simulink model "c00015M_harness"  (R2018a)
settings: Solver=FixedStepAuto  StartTime=0.0  StopTime=300  FixedStep=0.1  RelTol=1e-3
undefined symbols (not defined in the file): A1, hmax, PriorityTank, R1, R2, sigbuilder_block, TempThreshold
(part 9 of 33)

== system c00015M_harness/M078/Tank3 ==
  CT3 : Inport
  T3 : Inport  Port=2
  EB3 : Inport  Port=3
  LL1 : Inport  Port=4
  Control : Subsystem
  Logical Operator : Logic  AllPortsSameDT=off  OutDataTypeStr=boolean
  MasterTankControl : Subsystem
  Memory : Memory
  Memory1 : Memory
  TankModel : Subsystem
  LL3 : Outport
  wires:
  TankModel/1(LiquidLevel) -> Memory/1, LL3/1
  Control/1(LiquidIn) -> Logical Operator/1
  Control/2(LiquidOut) -> TankModel/2(LiquidOut)
  Memory/1 -> MasterTankControl/2(LiquidTank3), Control/5(LiquidLevel)
  CT3/1 -> Control/2(StartMaintenance), Control/1(ControlType)
  Memory1/1 -> MasterTankControl/1(LiquidTank1)
  EB3/1 -> Control/3(EmergencyButton)
  MasterTankControl/1(AllowTheTankFilling) -> Logical Operator/2
  Logical Operator/1 -> TankModel/1(LiquidIn)
  LL1/1 -> Memory1/1
  T3/1 -> Control/4(Temperature)

== system c00015M_harness/M079/Tank1 ==
  CT1 : Inport
  T1 : Inport  Port=2
  EB1 : Inport  Port=3
  LL3 : Inport  Port=4
  Control : Subsystem
  Logical Operator : Logic  AllPortsSameDT=off  OutDataTypeStr=boolean
  MasterTankControl : Subsystem
  Memory : Memory
  Memory2 : Memory
  TankModel : Subsystem
  LL1 : Outport
  wires:
  TankModel/1(LiquidLevel) -> Memory/1, LL1/1
  Control/1(LiquidIn) -> Logical Operator/1
  Control/2(LiquidOut) -> TankModel/2(LiquidOut)
  Memory/1 -> Control/5(LiquidLevel), MasterTankControl/1(LiquidTank1)
  CT1/1 -> Control/2(StartMaintenance), Control/1(ControlType)
  LL3/1 -> Memory2/1
  Memory2/1 -> MasterTankControl/2(LiquidTank3)
  EB1/1 -> Control/3(EmergencyButton)
  MasterTankControl/1(AllowTheTankFilling) -> Logical Operator/2
  Logical Operator/1 -> TankModel/1(LiquidIn)
  T1/1 -> Control/4(Temperature)

== system c00015M_harness/M079/Tank3 ==
  CT3 : Inport
  T3 : Inport  Port=2
  EB3 : Inport  Port=3
  LL1 : Inport  Port=4
  Control : Subsystem
  Logical Operator : Logic  AllPortsSameDT=off  OutDataTypeStr=boolean
  MasterTankControl : Subsystem
  Memory : Memory
  Memory1 : Memory
  TankModel : Subsystem
  LL3 : Outport
  wires:
  TankModel/1(LiquidLevel) -> Memory/1, LL3/1
  Control/1(LiquidIn) -> Logical Operator/1
  Control/2(LiquidOut) -> TankModel/2(LiquidOut)
  Memory/1 -> MasterTankControl/2(LiquidTank3), Control/5(LiquidLevel)
  CT3/1 -> Control/2(StartMaintenance), Control/1(ControlType)
  Memory1/1 -> MasterTankControl/1(LiquidTank1)
  EB3/1 -> Control/3(EmergencyButton)
  MasterTankControl/1(AllowTheTankFilling) -> Logical Operator/2
  Logical Operator/1 -> TankModel/1(LiquidIn)
  LL1/1 -> Memory1/1
  T3/1 -> Control/4(Temperature)

== system c00015M_harness/M080/Tank1 ==
  CT1 : Inport
  T1 : Inport  Port=2
  EB1 : Inport  Port=3
  LL3 : Inport  Port=4
  Control : Subsystem
  Logical Operator : Logic  AllPortsSameDT=off  OutDataTypeStr=boolean
  MasterTankControl : Subsystem
  Memory : Memory
  Memory2 : Memory
  TankModel : Subsystem
  LL1 : Outport
  wires:
  TankModel/1(LiquidLevel) -> Memory/1, LL1/1
  Control/1(LiquidIn) -> Logical Operator/1
  Control/2(LiquidOut) -> TankModel/2(LiquidOut)
  Memory/1 -> Control/5(LiquidLevel), MasterTankControl/1(LiquidTank1)
  CT1/1 -> Control/2(StartMaintenance), Control/1(ControlType)
  LL3/1 -> Memory2/1
  Memory2/1 -> MasterTankControl/2(LiquidTank3)
  EB1/1 -> Control/3(EmergencyButton)
  MasterTankControl/1(AllowTheTankFilling) -> Logical Operator/2
  Logical Operator/1 -> TankModel/1(LiquidIn)
  T1/1 -> Control/4(Temperature)

== system c00015M_harness/M080/Tank3 ==
  CT3 : Inport
  T3 : Inport  Port=2
  EB3 : Inport  Port=3
  LL1 : Inport  Port=4
  Control : Subsystem
  Logical Operator : Logic  AllPortsSameDT=off  OutDataTypeStr=boolean
  MasterTankControl : Subsystem
  Memory : Memory
  Memory1 : Memory
  TankModel : Subsystem
  LL3 : Outport
  wires:
  TankModel/1(LiquidLevel) -> Memory/1, LL3/1
  Control/1(LiquidIn) -> Logical Operator/1
  Control/2(LiquidOut) -> TankModel/2(LiquidOut)
  Memory/1 -> MasterTankControl/2(LiquidTank3), Control/5(LiquidLevel)
  CT3/1 -> Control/2(StartMaintenance), Control/1(ControlType)
  Memory1/1 -> MasterTankControl/1(LiquidTank1)
  EB3/1 -> Control/3(EmergencyButton)
  MasterTankControl/1(AllowTheTankFilling) -> Logical Operator/2
  Logical Operator/1 -> TankModel/1(LiquidIn)
  LL1/1 -> Memory1/1
  T3/1 -> Control/4(Temperature)

== system c00015M_harness/M081/Tank1 ==
  CT1 : Inport
  T1 : Inport  Port=2
  EB1 : Inport  Port=3
  LL3 : Inport  Port=4
  Control : Subsystem
  Logical Operator : Logic  AllPortsSameDT=off  OutDataTypeStr=boolean
  MasterTankControl : Subsystem
  Memory : Memory
  Memory2 : Memory
  TankModel : Subsystem
  LL1 : Outport
  wires:
  TankModel/1(LiquidLevel) -> Memory/1, LL1/1
  Control/1(LiquidIn) -> Logical Operator/1
  Control/2(LiquidOut) -> TankModel/2(LiquidOut)
  Memory/1 -> Control/5(LiquidLevel), MasterTankControl/1(LiquidTank1)
  CT1/1 -> Control/2(StartMaintenance), Control/1(ControlType)
  LL3/1 -> Memory2/1
  Memory2/1 -> MasterTankControl/2(LiquidTank3)
  EB1/1 -> Control/3(EmergencyButton)
  MasterTankControl/1(AllowTheTankFilling) -> Logical Operator/2
  Logical Operator/1 -> TankModel/1(LiquidIn)
  T1/1 -> Control/4(Temperature)

== system c00015M_harness/M081/Tank3 ==
  CT3 : Inport
  T3 : Inport  Port=2
  EB3 : Inport  Port=3
  LL1 : Inport  Port=4
  Control : Subsystem
  Logical Operator : Logic  AllPortsSameDT=off  OutDataTypeStr=boolean
  MasterTankControl : Subsystem
  Memory : Memory
  Memory1 : Memory
  TankModel : Subsystem
  LL3 : Outport
  wires:
  TankModel/1(LiquidLevel) -> Memory/1, LL3/1
  Control/1(LiquidIn) -> Logical Operator/1
  Control/2(LiquidOut) -> TankModel/2(LiquidOut)
  Memory/1 -> MasterTankControl/2(LiquidTank3), Control/5(LiquidLevel)
  CT3/1 -> Control/2(StartMaintenance), Control/1(ControlType)
  Memory1/1 -> MasterTankControl/1(LiquidTank1)
  EB3/1 -> Control/3(EmergencyButton)
  MasterTankControl/1(AllowTheTankFilling) -> Logical Operator/2
  Logical Operator/1 -> TankModel/1(LiquidIn)
  LL1/1 -> Memory1/1
  T3/1 -> Control/4(Temperature)

== system c00015M_harness/M082/Tank1 ==
  CT1 : Inport
  T1 : Inport  Port=2
  EB1 : Inport  Port=3
  LL3 : Inport  Port=4
  Control : Subsystem
  Logical Operator : Logic  AllPortsSameDT=off  OutDataTypeStr=boolean
  MasterTankControl : Subsystem
  Memory : Memory
  Memory2 : Memory
  TankModel : Subsystem
  LL1 : Outport
  wires:
  TankModel/1(LiquidLevel) -> Memory/1, LL1/1
  Control/1(LiquidIn) -> Logical Operator/1
  Control/2(LiquidOut) -> TankModel/2(LiquidOut)
  Memory/1 -> Control/5(LiquidLevel), MasterTankControl/1(LiquidTank1)
  CT1/1 -> Control/2(StartMaintenance), Control/1(ControlType)
  LL3/1 -> Memory2/1
  Memory2/1 -> MasterTankControl/2(LiquidTank3)
  EB1/1 -> Control/3(EmergencyButton)
  MasterTankControl/1(AllowTheTankFilling) -> Logical Operator/2
  Logical Operator/1 -> TankModel/1(LiquidIn)
  T1/1 -> Control/4(Temperature)

== system c00015M_harness/M082/Tank3 ==
  CT3 : Inport
  T3 : Inport  Port=2
  EB3 : Inport  Port=3
  LL1 : Inport  Port=4
  Control : Subsystem
  Logical Operator : Logic  AllPortsSameDT=off  OutDataTypeStr=boolean
  MasterTankControl : Subsystem
  Memory : Memory
  Memory1 : Memory
  TankModel : Subsystem
  LL3 : Outport
  wires:
  TankModel/1(LiquidLevel) -> Memory/1, LL3/1
  Control/1(LiquidIn) -> Logical Operator/1
  Control/2(LiquidOut) -> TankModel/2(LiquidOut)
  Memory/1 -> MasterTankControl/2(LiquidTank3), Control/5(LiquidLevel)
  CT3/1 -> Control/2(StartMaintenance), Control/1(ControlType)
  Memory1/1 -> MasterTankControl/1(LiquidTank1)
  EB3/1 -> Control/3(EmergencyButton)
  MasterTankControl/1(AllowTheTankFilling) -> Logical Operator/2
  Logical Operator/1 -> TankModel/1(LiquidIn)
  LL1/1 -> Memory1/1
  T3/1 -> Control/4(Temperature)

== system c00015M_harness/M144/Tank1 ==
  CT1 : Inport
  T1 : Inport  Port=2
  EB1 : Inport  Port=3
  LL3 : Inport  Port=4
  Control : Subsystem
  Logical Operator : Logic  AllPortsSameDT=off  OutDataTypeStr=boolean
  MasterTankControl : Subsystem
  Memory : Memory
  Memory2 : Memory
  TankModel : Subsystem
  LL1 : Outport
  wires:
  TankModel/1(LiquidLevel) -> Memory/1, LL1/1
  Control/1(LiquidIn) -> Logical Operator/1
  Control/2(LiquidOut) -> TankModel/2(LiquidOut)
  Memory/1 -> Control/5(LiquidLevel), MasterTankControl/1(LiquidTank1)
  CT1/1 -> Control/2(StartMaintenance), Control/1(ControlType)
  LL3/1 -> Memory2/1
  Memory2/1 -> MasterTankControl/2(LiquidTank3)
  EB1/1 -> Control/3(EmergencyButton)
  MasterTankControl/1(AllowTheTankFilling) -> Logical Operator/2
  Logical Operator/1 -> TankModel/1(LiquidIn)
  T1/1 -> Control/4(Temperature)

== system c00015M_harness/M144/Tank3 ==
  CT3 : Inport
  T3 : Inport  Port=2
  EB3 : Inport  Port=3
  LL1 : Inport  Port=4
  Control : Subsystem
  Logical Operator : Logic  AllPortsSameDT=off  OutDataTypeStr=boolean
  MasterTankControl : Subsystem
  Memory : Memory
  Memory1 : Memory
  TankModel : Subsystem
  LL3 : Outport
  wires:
  TankModel/1(LiquidLevel) -> Memory/1, LL3/1
  Control/1(LiquidIn) -> Logical Operator/1
  Control/2(LiquidOut) -> TankModel/2(LiquidOut)
  Memory/1 -> MasterTankControl/2(LiquidTank3), Control/5(LiquidLevel)
  CT3/1 -> Control/2(StartMaintenance), Control/1(ControlType)
  Memory1/1 -> MasterTankControl/1(LiquidTank1)
  EB3/1 -> Control/3(EmergencyButton)
  MasterTankControl/1(AllowTheTankFilling) -> Logical Operator/2
  Logical Operator/1 -> TankModel/1(LiquidIn)
  LL1/1 -> Memory1/1
  T3/1 -> Control/4(Temperature)

== system c00015M_harness/M145/Tank1 ==
  CT1 : Inport
  T1 : Inport  Port=2
  EB1 : Inport  Port=3
  LL3 : Inport  Port=4
  Control : Subsystem
  Logical Operator : Logic  AllPortsSameDT=off  OutDataTypeStr=boolean
  MasterTankControl : Subsystem
  Memory : Memory
  Memory2 : Memory
  TankModel : Subsystem
  LL1 : Outport
  wires:
  TankModel/1(LiquidLevel) -> Memory/1, LL1/1
  Control/1(LiquidIn) -> Logical Operator/1
  Control/2(LiquidOut) -> TankModel/2(LiquidOut)
  Memory/1 -> Control/5(LiquidLevel), MasterTankControl/1(LiquidTank1)
  CT1/1 -> Control/2(StartMaintenance), Control/1(ControlType)
  LL3/1 -> Memory2/1
  Memory2/1 -> MasterTankControl/2(LiquidTank3)
  EB1/1 -> Control/3(EmergencyButton)
  MasterTankControl/1(AllowTheTankFilling) -> Logical Operator/2
  Logical Operator/1 -> TankModel/1(LiquidIn)
  T1/1 -> Control/4(Temperature)

== system c00015M_harness/M145/Tank3 ==
  CT3 : Inport
  T3 : Inport  Port=2
  EB3 : Inport  Port=3
  LL1 : Inport  Port=4
  Control : Subsystem
  Logical Operator : Logic  AllPortsSameDT=off  OutDataTypeStr=boolean
  MasterTankControl : Subsystem
  Memory : Memory
  Memory1 : Memory
  TankModel : Subsystem
  LL3 : Outport
  wires:
  TankModel/1(LiquidLevel) -> Memory/1, LL3/1
  Control/1(LiquidIn) -> Logical Operator/1
  Control/2(LiquidOut) -> TankModel/2(LiquidOut)
  Memory/1 -> MasterTankControl/2(LiquidTank3), Control/5(LiquidLevel)
  CT3/1 -> Control/2(StartMaintenance), Control/1(ControlType)
  Memory1/1 -> MasterTankControl/1(LiquidTank1)
  EB3/1 -> Control/3(EmergencyButton)
  MasterTankControl/1(AllowTheTankFilling) -> Logical Operator/2
  Logical Operator/1 -> TankModel/1(LiquidIn)
  LL1/1 -> Memory1/1
  T3/1 -> Control/4(Temperature)

== system c00015M_harness/M146/Tank1 ==
  CT1 : Inport
  T1 : Inport  Port=2
  EB1 : Inport  Port=3
  LL3 : Inport  Port=4
  Control : Subsystem
  Logical Operator : Logic  AllPortsSameDT=off  OutDataTypeStr=boolean
  MasterTankControl : Subsystem
  Memory : Memory
  Memory2 : Memory
  TankModel : Subsystem
  LL1 : Outport
  wires:
  TankModel/1(LiquidLevel) -> Memory/1, LL1/1
  Control/1(LiquidIn) -> Logical Operator/1
  Control/2(LiquidOut) -> TankModel/2(LiquidOut)
  Memory/1 -> Control/5(LiquidLevel), MasterTankControl/1(LiquidTank1)
  CT1/1 -> Control/2(StartMaintenance), Control/1(ControlType)
  LL3/1 -> Memory2/1
  Memory2/1 -> MasterTankControl/2(LiquidTank3)
  EB1/1 -> Control/3(EmergencyButton)
  MasterTankControl/1(AllowTheTankFilling) -> Logical Operator/2
  Logical Operator/1 -> TankModel/1(LiquidIn)
  T1/1 -> Control/4(Temperature)

== system c00015M_harness/M146/Tank3 ==
  CT3 : Inport
  T3 : Inport  Port=2
  EB3 : Inport  Port=3
  LL1 : Inport  Port=4
  Control : Subsystem
  Logical Operator : Logic  AllPortsSameDT=off  OutDataTypeStr=boolean
  MasterTankControl : Subsystem
  Memory : Memory
  Memory1 : Memory
  TankModel : Subsystem
  LL3 : Outport
  wires:
  TankModel/1(LiquidLevel) -> Memory/1, LL3/1
  Control/1(LiquidIn) -> Logical Operator/1
  Control/2(LiquidOut) -> TankModel/2(LiquidOut)
  Memory/1 -> MasterTankControl/2(LiquidTank3), Control/5(LiquidLevel)
  CT3/1 -> Control/2(StartMaintenance), Control/1(ControlType)
  Memory1/1 -> MasterTankControl/1(LiquidTank1)
  EB3/1 -> Control/3(EmergencyButton)
  MasterTankControl/1(AllowTheTankFilling) -> Logical Operator/2
  Logical Operator/1 -> TankModel/1(LiquidIn)
  LL1/1 -> Memory1/1
  T3/1 -> Control/4(Temperature)

== system c00015M_harness/M147/Tank1 ==
  CT1 : Inport
  T1 : Inport  Port=2
  EB1 : Inport  Port=3
  LL3 : Inport  Port=4
  Control : Subsystem
  Logical Operator : Logic  AllPortsSameDT=off  OutDataTypeStr=boolean
  MasterTankControl : Subsystem
  Memory : Memory
  Memory2 : Memory
  TankModel : Subsystem
  LL1 : Outport
  wires:
  TankModel/1(LiquidLevel) -> Memory/1, LL1/1
  Control/1(LiquidIn) -> Logical Operator/1
  Control/2(LiquidOut) -> TankModel/2(LiquidOut)
  Memory/1 -> Control/5(LiquidLevel), MasterTankControl/1(LiquidTank1)
  CT1/1 -> Control/2(StartMaintenance), Control/1(ControlType)
  LL3/1 -> Memory2/1
  Memory2/1 -> MasterTankControl/2(LiquidTank3)
  EB1/1 -> Control/3(EmergencyButton)
  MasterTankControl/1(AllowTheTankFilling) -> Logical Operator/2
  Logical Operator/1 -> TankModel/1(LiquidIn)
  T1/1 -> Control/4(Temperature)

== system c00015M_harness/M147/Tank3 ==
  CT3 : Inport
  T3 : Inport  Port=2
  EB3 : Inport  Port=3
  LL1 : Inport  Port=4
  Control : Subsystem
  Logical Operator : Logic  AllPortsSameDT=off  OutDataTypeStr=boolean
  MasterTankControl : Subsystem
  Memory : Memory
  Memory1 : Memory
  TankModel : Subsystem
  LL3 : Outport
  wires:
  TankModel/1(LiquidLevel) -> Memory/1, LL3/1
  Control/1(LiquidIn) -> Logical Operator/1
  Control/2(LiquidOut) -> TankModel/2(LiquidOut)
  Memory/1 -> MasterTankControl/2(LiquidTank3), Control/5(LiquidLevel)
  CT3/1 -> Control/2(StartMaintenance), Control/1(ControlType)
  Memory1/1 -> MasterTankControl/1(LiquidTank1)
  EB3/1 -> Control/3(EmergencyButton)
  MasterTankControl/1(AllowTheTankFilling) -> Logical Operator/2
  Logical Operator/1 -> TankModel/1(LiquidIn)
  LL1/1 -> Memory1/1
  T3/1 -> Control/4(Temperature)

== system c00015M_harness/M148/Tank1 ==
  CT1 : Inport
  T1 : Inport  Port=2
  EB1 : Inport  Port=3
  LL3 : Inport  Port=4
  Control : Subsystem
  Logical Operator : Logic  AllPortsSameDT=off  OutDataTypeStr=boolean
  MasterTankControl : Subsystem
  Memory : Memory
  Memory2 : Memory
  TankModel : Subsystem
  LL1 : Outport
  wires:
  TankModel/1(LiquidLevel) -> Memory/1, LL1/1
  Control/1(LiquidIn) -> Logical Operator/1
  Control/2(LiquidOut) -> TankModel/2(LiquidOut)
  Memory/1 -> Control/5(LiquidLevel), MasterTankControl/1(LiquidTank1)
  CT1/1 -> Control/2(StartMaintenance), Control/1(ControlType)
  LL3/1 -> Memory2/1
  Memory2/1 -> MasterTankControl/2(LiquidTank3)
  EB1/1 -> Control/3(EmergencyButton)
  MasterTankControl/1(AllowTheTankFilling) -> Logical Operator/2
  Logical Operator/1 -> TankModel/1(LiquidIn)
  T1/1 -> Control/4(Temperature)

== system c00015M_harness/M148/Tank3 ==
  CT3 : Inport
  T3 : Inport  Port=2
  EB3 : Inport  Port=3
  LL1 : Inport  Port=4
  Control : Subsystem
  Logical Operator : Logic  AllPortsSameDT=off  OutDataTypeStr=boolean
  MasterTankControl : Subsystem
  Memory : Memory
  Memory1 : Memory
  TankModel : Subsystem
  LL3 : Outport
  wires:
  TankModel/1(LiquidLevel) -> Memory/1, LL3/1
  Control/1(LiquidIn) -> Logical Operator/1
  Control/2(LiquidOut) -> TankModel/2(LiquidOut)
  Memory/1 -> MasterTankControl/2(LiquidTank3), Control/5(LiquidLevel)
  CT3/1 -> Control/2(StartMaintenance), Control/1(ControlType)
  Memory1/1 -> MasterTankControl/1(LiquidTank1)
  EB3/1 -> Control/3(EmergencyButton)
  MasterTankControl/1(AllowTheTankFilling) -> Logical Operator/2
  Logical Operator/1 -> TankModel/1(LiquidIn)
  LL1/1 -> Memory1/1
  T3/1 -> Control/4(Temperature)

== system c00015M_harness/M165/Tank1 ==
  CT1 : Inport
  T1 : Inport  Port=2
  EB1 : Inport  Port=3
  LL3 : Inport  Port=4
  Control : Subsystem
  Logical Operator : Logic  AllPortsSameDT=off  OutDataTypeStr=boolean
  MasterTankControl : Subsystem
  Memory : Memory
  Memory2 : Memory
  TankModel : Subsystem
  LL1 : Outport
  wires:
  TankModel/1(LiquidLevel) -> Memory/1, LL1/1
  Control/1(LiquidIn) -> Logical Operator/1
  Control/2(LiquidOut) -> TankModel/2(LiquidOut)
  Memory/1 -> Control/5(LiquidLevel), MasterTankControl/1(LiquidTank1)
  CT1/1 -> Control/2(StartMaintenance), Control/1(ControlType)
  LL3/1 -> Memory2/1
  Memory2/1 -> MasterTankControl/2(LiquidTank3)
  EB1/1 -> Control/3(EmergencyButton)
  MasterTankControl/1(AllowTheTankFilling) -> Logical Operator/2
  Logical Operator/1 -> TankModel/1(LiquidIn)
  T1/1 -> Control/4(Temperature)

== system c00015M_harness/M165/Tank3 ==
  CT3 : Inport
  T3 : Inport  Port=2
  EB3 : Inport  Port=3
  LL1 : Inport  Port=4
  Control : Subsystem
  Logical Operator : Logic  AllPortsSameDT=off  OutDataTypeStr=boolean
  MasterTankControl : Subsystem
  Memory : Memory
  Memory1 : Memory
  TankModel : Subsystem
  LL3 : Outport
  wires:
  TankModel/1(LiquidLevel) -> Memory/1, LL3/1
  Control/1(LiquidIn) -> Logical Operator/1
  Control/2(LiquidOut) -> TankModel/2(LiquidOut)
  Memory/1 -> MasterTankControl/2(LiquidTank3), Control/5(LiquidLevel)
  CT3/1 -> Control/2(StartMaintenance), Control/1(ControlType)
  Memory1/1 -> MasterTankControl/1(LiquidTank1)
  EB3/1 -> Control/3(EmergencyButton)
  MasterTankControl/1(AllowTheTankFilling) -> Logical Operator/2
  Logical Operator/1 -> TankModel/1(LiquidIn)
  LL1/1 -> Memory1/1
  T3/1 -> Control/4(Temperature)

== system c00015M_harness/M166/Tank1 ==
  CT1 : Inport
  T1 : Inport  Port=2
  EB1 : Inport  Port=3
  LL3 : Inport  Port=4
  Control : Subsystem
  Logical Operator : Logic  AllPortsSameDT=off  OutDataTypeStr=boolean
  MasterTankControl : Subsystem
  Memory : Memory
  Memory2 : Memory
  TankModel : Subsystem
  LL1 : Outport
  wires:
  TankModel/1(LiquidLevel) -> Memory/1, LL1/1
  Control/1(LiquidIn) -> Logical Operator/1
  Control/2(LiquidOut) -> TankModel/2(LiquidOut)
  Memory/1 -> Control/5(LiquidLevel), MasterTankControl/1(LiquidTank1)
  CT1/1 -> Control/2(StartMaintenance), Control/1(ControlType)
  LL3/1 -> Memory2/1
  Memory2/1 -> MasterTankControl/2(LiquidTank3)
  EB1/1 -> Control/3(EmergencyButton)
  MasterTankControl/1(AllowTheTankFilling) -> Logical Operator/2
  Logical Operator/1 -> TankModel/1(LiquidIn)
  T1/1 -> Control/4(Temperature)

== system c00015M_harness/M166/Tank3 ==
  CT3 : Inport
  T3 : Inport  Port=2
  EB3 : Inport  Port=3
  LL1 : Inport  Port=4
  Control : Subsystem
  Logical Operator : Logic  AllPortsSameDT=off  OutDataTypeStr=boolean
  MasterTankControl : Subsystem
  Memory : Memory
  Memory1 : Memory
  TankModel : Subsystem
  LL3 : Outport
  wires:
  TankModel/1(LiquidLevel) -> Memory/1, LL3/1
  Control/1(LiquidIn) -> Logical Operator/1
  Control/2(LiquidOut) -> TankModel/2(LiquidOut)
  Memory/1 -> MasterTankControl/2(LiquidTank3), Control/5(LiquidLevel)
  CT3/1 -> Control/2(StartMaintenance), Control/1(ControlType)
  Memory1/1 -> MasterTankControl/1(LiquidTank1)
  EB3/1 -> Control/3(EmergencyButton)
  MasterTankControl/1(AllowTheTankFilling) -> Logical Operator/2
  Logical Operator/1 -> TankModel/1(LiquidIn)
  LL1/1 -> Memory1/1
  T3/1 -> Control/4(Temperature)

== system c00015M_harness/M167/Tank1 ==
  CT1 : Inport
  T1 : Inport  Port=2
  EB1 : Inport  Port=3
  LL3 : Inport  Port=4
  Control : Subsystem
  Logical Operator : Logic  AllPortsSameDT=off  OutDataTypeStr=boolean
  MasterTankControl : Subsystem
  Memory : Memory
  Memory2 : Memory
  TankModel : Subsystem
  LL1 : Outport
  wires:
  TankModel/1(LiquidLevel) -> Memory/1, LL1/1
  Control/1(LiquidIn) -> Logical Operator/1
  Control/2(LiquidOut) -> TankModel/2(LiquidOut)
  Memory/1 -> Control/5(LiquidLevel), MasterTankControl/1(LiquidTank1)
  CT1/1 -> Control/2(StartMaintenance), Control/1(ControlType)
  LL3/1 -> Memory2/1
  Memory2/1 -> MasterTankControl/2(LiquidTank3)
  EB1/1 -> Control/3(EmergencyButton)
  MasterTankControl/1(AllowTheTankFilling) -> Logical Operator/2
  Logical Operator/1 -> TankModel/1(LiquidIn)
  T1/1 -> Control/4(Temperature)

== system c00015M_harness/M167/Tank3 ==
  CT3 : Inport
  T3 : Inport  Port=2
  EB3 : Inport  Port=3
  LL1 : Inport  Port=4
  Control : Subsystem
  Logical Operator : Logic  AllPortsSameDT=off  OutDataTypeStr=boolean
  MasterTankControl : Subsystem
  Memory : Memory
  Memory1 : Memory
  TankModel : Subsystem
  LL3 : Outport
  wires:
  TankModel/1(LiquidLevel) -> Memory/1, LL3/1
  Control/1(LiquidIn) -> Logical Operator/1
  Control/2(LiquidOut) -> TankModel/2(LiquidOut)
  Memory/1 -> MasterTankControl/2(LiquidTank3), Control/5(LiquidLevel)
  CT3/1 -> Control/2(StartMaintenance), Control/1(ControlType)
  Memory1/1 -> MasterTankControl/1(LiquidTank1)
  EB3/1 -> Control/3(EmergencyButton)
  MasterTankControl/1(AllowTheTankFilling) -> Logical Operator/2
  Logical Operator/1 -> TankModel/1(LiquidIn)
  LL1/1 -> Memory1/1
  T3/1 -> Control/4(Temperature)

== system c00015M_harness/M168/Tank1 ==
  CT1 : Inport
  T1 : Inport  Port=2
  EB1 : Inport  Port=3
  LL3 : Inport  Port=4
  Control : Subsystem
  Logical Operator : Logic  AllPortsSameDT=off  OutDataTypeStr=boolean
  MasterTankControl : Subsystem
  Memory : Memory
  Memory2 : Memory
  TankModel : Subsystem
  LL1 : Outport
  wires:
  TankModel/1(LiquidLevel) -> Memory/1, LL1/1
  Control/1(LiquidIn) -> Logical Operator/1
  Control/2(LiquidOut) -> TankModel/2(LiquidOut)
  Memory/1 -> Control/5(LiquidLevel), MasterTankControl/1(LiquidTank1)
  CT1/1 -> Control/2(StartMaintenance), Control/1(ControlType)
  LL3/1 -> Memory2/1
  Memory2/1 -> MasterTankControl/2(LiquidTank3)
  EB1/1 -> Control/3(EmergencyButton)
  MasterTankControl/1(AllowTheTankFilling) -> Logical Operator/2
  Logical Operator/1 -> TankModel/1(LiquidIn)
  T1/1 -> Control/4(Temperature)

== system c00015M_harness/M168/Tank3 ==
  CT3 : Inport
  T3 : Inport  Port=2
  EB3 : Inport  Port=3
  LL1 : Inport  Port=4
  Control : Subsystem
  Logical Operator : Logic  AllPortsSameDT=off  OutDataTypeStr=boolean
  MasterTankControl : Subsystem
  Memory : Memory
  Memory1 : Memory
  TankModel : Subsystem
  LL3 : Outport
  wires:
  TankModel/1(LiquidLevel) -> Memory/1, LL3/1
  Control/1(LiquidIn) -> Logical Operator/1
  Control/2(LiquidOut) -> TankModel/2(LiquidOut)
  Memory/1 -> MasterTankControl/2(LiquidTank3), Control/5(LiquidLevel)
  CT3/1 -> Control/2(StartMaintenance), Control/1(ControlType)
  Memory1/1 -> MasterTankControl/1(LiquidTank1)
  EB3/1 -> Control/3(EmergencyButton)
  MasterTankControl/1(AllowTheTankFilling) -> Logical Operator/2
  Logical Operator/1 -> TankModel/1(LiquidIn)
  LL1/1 -> Memory1/1
  T3/1 -> Control/4(Temperature)

== system c00015M_harness/M169/Tank1 ==
  CT1 : Inport
  T1 : Inport  Port=2
  EB1 : Inport  Port=3
  LL3 : Inport  Port=4
  Control : Subsystem
  Logical Operator : Logic  AllPortsSameDT=off  OutDataTypeStr=boolean
  MasterTankControl : Subsystem
  Memory : Memory
  Memory2 : Memory
  TankModel : Subsystem
  LL1 : Outport
  wires:
  TankModel/1(LiquidLevel) -> Memory/1, LL1/1
  Control/1(LiquidIn) -> Logical Operator/1
  Control/2(LiquidOut) -> TankModel/2(LiquidOut)
  Memory/1 -> Control/5(LiquidLevel), MasterTankControl/1(LiquidTank1)
  CT1/1 -> Control/2(StartMaintenance), Control/1(ControlType)
  LL3/1 -> Memory2/1
  Memory2/1 -> MasterTankControl/2(LiquidTank3)
  EB1/1 -> Control/3(EmergencyButton)
  MasterTankControl/1(AllowTheTankFilling) -> Logical Operator/2
  Logical Operator/1 -> TankModel/1(LiquidIn)
  T1/1 -> Control/4(Temperature)

== system c00015M_harness/M169/Tank3 ==
  CT3 : Inport
  T3 : Inport  Port=2
  EB3 : Inport  Port=3
  LL1 : Inport  Port=4
  Control : Subsystem
  Logical Operator : Logic  AllPortsSameDT=off  OutDataTypeStr=boolean
  MasterTankControl : Subsystem
  Memory : Memory
  Memory1 : Memory
  TankModel : Subsystem
  LL3 : Outport
  wires:
  TankModel/1(LiquidLevel) -> Memory/1, LL3/1
  Control/1(LiquidIn) -> Logical Operator/1
  Control/2(LiquidOut) -> TankModel/2(LiquidOut)
  Memory/1 -> MasterTankControl/2(LiquidTank3), Control/5(LiquidLevel)
  CT3/1 -> Control/2(StartMaintenance), Control/1(ControlType)
  Memory1/1 -> MasterTankControl/1(LiquidTank1)
  EB3/1 -> Control/3(EmergencyButton)
  MasterTankControl/1(AllowTheTankFilling) -> Logical Operator/2
  Logical Operator/1 -> TankModel/1(LiquidIn)
  LL1/1 -> Memory1/1
  T3/1 -> Control/4(Temperature)

== system c00015M_harness/M170/Tank1 ==
  CT1 : Inport
  T1 : Inport  Port=2
  EB1 : Inport  Port=3
  LL3 : Inport  Port=4
  Control : Subsystem
  Logical Operator : Logic  AllPortsSameDT=off  OutDataTypeStr=boolean
  MasterTankControl : Subsystem
  Memory : Memory
  Memory2 : Memory
  TankModel : Subsystem
  LL1 : Outport
  wires:
  TankModel/1(LiquidLevel) -> Memory/1, LL1/1
  Control/1(LiquidIn) -> Logical Operator/1
  Control/2(LiquidOut) -> TankModel/2(LiquidOut)
  Memory/1 -> Control/5(LiquidLevel), MasterTankControl/1(LiquidTank1)
  CT1/1 -> Control/2(StartMaintenance), Control/1(ControlType)
  LL3/1 -> Memory2/1
  Memory2/1 -> MasterTankControl/2(LiquidTank3)
  EB1/1 -> Control/3(EmergencyButton)
  MasterTankControl/1(AllowTheTankFilling) -> Logical Operator/2
  Logical Operator/1 -> TankModel/1(LiquidIn)
  T1/1 -> Control/4(Temperature)

== system c00015M_harness/M170/Tank3 ==
  CT3 : Inport
  T3 : Inport  Port=2
  EB3 : Inport  Port=3
  LL1 : Inport  Port=4
  Control : Subsystem
  Logical Operator : Logic  AllPortsSameDT=off  OutDataTypeStr=boolean
  MasterTankControl : Subsystem
  Memory : Memory
  Memory1 : Memory
  TankModel : Subsystem
  LL3 : Outport
  wires:
  TankModel/1(LiquidLevel) -> Memory/1, LL3/1
  Control/1(LiquidIn) -> Logical Operator/1
  Control/2(LiquidOut) -> TankModel/2(LiquidOut)
  Memory/1 -> MasterTankControl/2(LiquidTank3), Control/5(LiquidLevel)
  CT3/1 -> Control/2(StartMaintenance), Control/1(ControlType)
  Memory1/1 -> MasterTankControl/1(LiquidTank1)
  EB3/1 -> Control/3(EmergencyButton)
  MasterTankControl/1(AllowTheTankFilling) -> Logical Operator/2
  Logical Operator/1 -> TankModel/1(LiquidIn)
  LL1/1 -> Memory1/1
  T3/1 -> Control/4(Temperature)

== system c00015M_harness/M171/Tank1 ==
  CT1 : Inport
  T1 : Inport  Port=2
  EB1 : Inport  Port=3
  LL3 : Inport  Port=4
  Control : Subsystem
  Logical Operator : Logic  AllPortsSameDT=off  OutDataTypeStr=boolean
  MasterTankControl : Subsystem
  Memory : Memory
  Memory2 : Memory
  TankModel : Subsystem
  LL1 : Outport
  wires:
  TankModel/1(LiquidLevel) -> Memory/1, LL1/1
  Control/1(LiquidIn) -> Logical Operator/1
  Control/2(LiquidOut) -> TankModel/2(LiquidOut)
  Memory/1 -> Control/5(LiquidLevel), MasterTankControl/1(LiquidTank1)
  CT1/1 -> Control/2(StartMaintenance), Control/1(ControlType)
  LL3/1 -> Memory2/1
  Memory2/1 -> MasterTankControl/2(LiquidTank3)
  EB1/1 -> Control/3(EmergencyButton)
  MasterTankControl/1(AllowTheTankFilling) -> Logical Operator/2
  Logical Operator/1 -> TankModel/1(LiquidIn)
  T1/1 -> Control/4(Temperature)

== system c00015M_harness/M171/Tank3 ==
  CT3 : Inport
  T3 : Inport  Port=2
  EB3 : Inport  Port=3
  LL1 : Inport  Port=4
  Control : Subsystem
  Logical Operator : Logic  AllPortsSameDT=off  OutDataTypeStr=boolean
  MasterTankControl : Subsystem
  Memory : Memory
  Memory1 : Memory
  TankModel : Subsystem
  LL3 : Outport
  wires:
  TankModel/1(LiquidLevel) -> Memory/1, LL3/1
  Control/1(LiquidIn) -> Logical Operator/1
  Control/2(LiquidOut) -> TankModel/2(LiquidOut)
  Memory/1 -> MasterTankControl/2(LiquidTank3), Control/5(LiquidLevel)
  CT3/1 -> Control/2(StartMaintenance), Control/1(ControlType)
  Memory1/1 -> MasterTankControl/1(LiquidTank1)
  EB3/1 -> Control/3(EmergencyButton)
  MasterTankControl/1(AllowTheTankFilling) -> Logical Operator/2
  Logical Operator/1 -> TankModel/1(LiquidIn)
  LL1/1 -> Memory1/1
  T3/1 -> Control/4(Temperature)

== system c00015M_harness/M172/Tank1 ==
  CT1 : Inport
  T1 : Inport  Port=2
  EB1 : Inport  Port=3
  LL3 : Inport  Port=4
  Control : Subsystem
  Logical Operator : Logic  AllPortsSameDT=off  OutDataTypeStr=boolean
  MasterTankControl : Subsystem
  Memory : Memory
  Memory2 : Memory
  TankModel : Subsystem
  LL1 : Outport
  wires:
  TankModel/1(LiquidLevel) -> Memory/1, LL1/1
  Control/1(LiquidIn) -> Logical Operator/1
  Control/2(LiquidOut) -> TankModel/2(LiquidOut)
  Memory/1 -> Control/5(LiquidLevel), MasterTankControl/1(LiquidTank1)
  CT1/1 -> Control/2(StartMaintenance), Control/1(ControlType)
  LL3/1 -> Memory2/1
  Memory2/1 -> MasterTankControl/2(LiquidTank3)
  EB1/1 -> Control/3(EmergencyButton)
  MasterTankControl/1(AllowTheTankFilling) -> Logical Operator/2
  Logical Operator/1 -> TankModel/1(LiquidIn)
  T1/1 -> Control/4(Temperature)

== system c00015M_harness/M172/Tank3 ==
  CT3 : Inport
  T3 : Inport  Port=2
  EB3 : Inport  Port=3
  LL1 : Inport  Port=4
  Control : Subsystem
  Logical Operator : Logic  AllPortsSameDT=off  OutDataTypeStr=boolean
  MasterTankControl : Subsystem
  Memory : Memory
  Memory1 : Memory
  TankModel : Subsystem
  LL3 : Outport
  wires:
  TankModel/1(LiquidLevel) -> Memory/1, LL3/1
  Control/1(LiquidIn) -> Logical Operator/1
  Control/2(LiquidOut) -> TankModel/2(LiquidOut)
  Memory/1 -> MasterTankControl/2(LiquidTank3), Control/5(LiquidLevel)
  CT3/1 -> Control/2(StartMaintenance), Control/1(ControlType)
  Memory1/1 -> MasterTankControl/1(LiquidTank1)
  EB3/1 -> Control/3(EmergencyButton)
  MasterTankControl/1(AllowTheTankFilling) -> Logical Operator/2
  Logical Operator/1 -> TankModel/1(LiquidIn)
  LL1/1 -> Memory1/1
  T3/1 -> Control/4(Temperature)

== system c00015M_harness/M173/Tank1 ==
  CT1 : Inport
  T1 : Inport  Port=2
  EB1 : Inport  Port=3
  LL3 : Inport  Port=4
  Control : Subsystem
  Logical Operator : Logic  AllPortsSameDT=off  OutDataTypeStr=boolean
  MasterTankControl : Subsystem
  Memory : Memory
  Memory2 : Memory
  TankModel : Subsystem
  LL1 : Outport
  wires:
  TankModel/1(LiquidLevel) -> Memory/1, LL1/1
  Control/1(LiquidIn) -> Logical Operator/1
  Control/2(LiquidOut) -> TankModel/2(LiquidOut)
  Memory/1 -> Control/5(LiquidLevel), MasterTankControl/1(LiquidTank1)
  CT1/1 -> Control/2(StartMaintenance), Control/1(ControlType)
  LL3/1 -> Memory2/1
  Memory2/1 -> MasterTankControl/2(LiquidTank3)
  EB1/1 -> Control/3(EmergencyButton)
  MasterTankControl/1(AllowTheTankFilling) -> Logical Operator/2
  Logical Operator/1 -> TankModel/1(LiquidIn)
  T1/1 -> Control/4(Temperature)

== system c00015M_harness/M173/Tank3 ==
  CT3 : Inport
  T3 : Inport  Port=2
  EB3 : Inport  Port=3
  LL1 : Inport  Port=4
  Control : Subsystem
  Logical Operator : Logic  AllPortsSameDT=off  OutDataTypeStr=boolean
  MasterTankControl : Subsystem
  Memory : Memory
  Memory1 : Memory
  TankModel : Subsystem
  LL3 : Outport
  wires:
  TankModel/1(LiquidLevel) -> Memory/1, LL3/1
  Control/1(LiquidIn) -> Logical Operator/1
  Control/2(LiquidOut) -> TankModel/2(LiquidOut)
  Memory/1 -> MasterTankControl/2(LiquidTank3), Control/5(LiquidLevel)
  CT3/1 -> Control/2(StartMaintenance), Control/1(ControlType)
  Memory1/1 -> MasterTankControl/1(LiquidTank1)
  EB3/1 -> Control/3(EmergencyButton)
  MasterTankControl/1(AllowTheTankFilling) -> Logical Operator/2
  Logical Operator/1 -> TankModel/1(LiquidIn)
  LL1/1 -> Memory1/1
  T3/1 -> Control/4(Temperature)

== system c00015M_harness/M174/Tank1 ==
  CT1 : Inport
  T1 : Inport  Port=2
  EB1 : Inport  Port=3
  LL3 : Inport  Port=4
  Control : Subsystem
  Logical Operator : Logic  AllPortsSameDT=off  OutDataTypeStr=boolean
  MasterTankControl : Subsystem
  Memory : Memory
  Memory2 : Memory
  TankModel : Subsystem
  LL1 : Outport
  wires:
  TankModel/1(LiquidLevel) -> Memory/1, LL1/1
  Control/1(LiquidIn) -> Logical Operator/1
  Control/2(LiquidOut) -> TankModel/2(LiquidOut)
  Memory/1 -> Control/5(LiquidLevel), MasterTankControl/1(LiquidTank1)
  CT1/1 -> Control/2(StartMaintenance), Control/1(ControlType)
  LL3/1 -> Memory2/1
  Memory2/1 -> MasterTankControl/2(LiquidTank3)
  EB1/1 -> Control/3(EmergencyButton)
  MasterTankControl/1(AllowTheTankFilling) -> Logical Operator/2
  Logical Operator/1 -> TankModel/1(LiquidIn)
  T1/1 -> Control/4(Temperature)

== system c00015M_harness/M174/Tank3 ==
  CT3 : Inport
  T3 : Inport  Port=2
  EB3 : Inport  Port=3
  LL1 : Inport  Port=4
  Control : Subsystem
  Logical Operator : Logic  AllPortsSameDT=off  OutDataTypeStr=boolean
  MasterTankControl : Subsystem
  Memory : Memory
  Memory1 : Memory
  TankModel : Subsystem
  LL3 : Outport
  wires:
  TankModel/1(LiquidLevel) -> Memory/1, LL3/1
  Control/1(LiquidIn) -> Logical Operator/1
  Control/2(LiquidOut) -> TankModel/2(LiquidOut)
  Memory/1 -> MasterTankControl/2(LiquidTank3), Control/5(LiquidLevel)
  CT3/1 -> Control/2(StartMaintenance), Control/1(ControlType)
  Memory1/1 -> MasterTankControl/1(LiquidTank1)
  EB3/1 -> Control/3(EmergencyButton)
  MasterTankControl/1(AllowTheTankFilling) -> Logical Operator/2
  Logical Operator/1 -> TankModel/1(LiquidIn)
  LL1/1 -> Memory1/1
  T3/1 -> Control/4(Temperature)

== system c00015M_harness/M175/Tank1 ==
  CT1 : Inport
  T1 : Inport  Port=2
  EB1 : Inport  Port=3
  LL3 : Inport  Port=4
  Control : Subsystem
  Logical Operator : Logic  AllPortsSameDT=off  OutDataTypeStr=boolean
  MasterTankControl : Subsystem
  Memory : Memory
  Memory2 : Memory
  TankModel : Subsystem
  LL1 : Outport
  wires:
  TankModel/1(LiquidLevel) -> Memory/1, LL1/1
  Control/1(LiquidIn) -> Logical Operator/1
  Control/2(LiquidOut) -> TankModel/2(LiquidOut)
  Memory/1 -> Control/5(LiquidLevel), MasterTankControl/1(LiquidTank1)
  CT1/1 -> Control/2(StartMaintenance), Control/1(ControlType)
  LL3/1 -> Memory2/1
  Memory2/1 -> MasterTankControl/2(LiquidTank3)
  EB1/1 -> Control/3(EmergencyButton)
  MasterTankControl/1(AllowTheTankFilling) -> Logical Operator/2
  Logical Operator/1 -> TankModel/1(LiquidIn)
  T1/1 -> Control/4(Temperature)

== system c00015M_harness/M175/Tank3 ==
  CT3 : Inport
  T3 : Inport  Port=2
  EB3 : Inport  Port=3
  LL1 : Inport  Port=4
  Control : Subsystem
  Logical Operator : Logic  AllPortsSameDT=off  OutDataTypeStr=boolean
  MasterTankControl : Subsystem
  Memory : Memory
  Memory1 : Memory
  TankModel : Subsystem
  LL3 : Outport
  wires:
  TankModel/1(LiquidLevel) -> Memory/1, LL3/1
  Control/1(LiquidIn) -> Logical Operator/1
  Control/2(LiquidOut) -> TankModel/2(LiquidOut)
  Memory/1 -> MasterTankControl/2(LiquidTank3), Control/5(LiquidLevel)
  CT3/1 -> Control/2(StartMaintenance), Control/1(ControlType)
  Memory1/1 -> MasterTankControl/1(LiquidTank1)
  EB3/1 -> Control/3(EmergencyButton)
  MasterTankControl/1(AllowTheTankFilling) -> Logical Operator/2
  Logical Operator/1 -> TankModel/1(LiquidIn)
  LL1/1 -> Memory1/1
  T3/1 -> Control/4(Temperature)

== system c00015M_harness/M176/Tank1 ==
  CT1 : Inport
  T1 : Inport  Port=2
  EB1 : Inport  Port=3
  LL3 : Inport  Port=4
  Control : Subsystem
  Logical Operator : Logic  AllPortsSameDT=off  OutDataTypeStr=boolean
  MasterTankControl : Subsystem
  Memory : Memory
  Memory2 : Memory
  TankModel : Subsystem
  LL1 : Outport
  wires:
  TankModel/1(LiquidLevel) -> Memory/1, LL1/1
  Control/1(LiquidIn) -> Logical Operator/1
  Control/2(LiquidOut) -> TankModel/2(LiquidOut)
  Memory/1 -> Control/5(LiquidLevel), MasterTankControl/1(LiquidTank1)
  CT1/1 -> Control/2(StartMaintenance), Control/1(ControlType)
  LL3/1 -> Memory2/1
  Memory2/1 -> MasterTankControl/2(LiquidTank3)
  EB1/1 -> Control/3(EmergencyButton)
  MasterTankControl/1(AllowTheTankFilling) -> Logical Operator/2
  Logical Operator/1 -> TankModel/1(LiquidIn)
  T1/1 -> Control/4(Temperature)

== system c00015M_harness/M176/Tank3 ==
  CT3 : Inport
  T3 : Inport  Port=2
  EB3 : Inport  Port=3
  LL1 : Inport  Port=4
  Control : Subsystem
  Logical Operator : Logic  AllPortsSameDT=off  OutDataTypeStr=boolean
  MasterTankControl : Subsystem
  Memory : Memory
  Memory1 : Memory
  TankModel : Subsystem
  LL3 : Outport
  wires:
  TankModel/1(LiquidLevel) -> Memory/1, LL3/1
  Control/1(LiquidIn) -> Logical Operator/1
  Control/2(LiquidOut) -> TankModel/2(LiquidOut)
  Memory/1 -> MasterTankControl/2(LiquidTank3), Control/5(LiquidLevel)
  CT3/1 -> Control/2(StartMaintenance), Control/1(ControlType)
  Memory1/1 -> MasterTankControl/1(LiquidTank1)
  EB3/1 -> Control/3(EmergencyButton)
  MasterTankControl/1(AllowTheTankFilling) -> Logical Operator/2
  Logical Operator/1 -> TankModel/1(LiquidIn)
  LL1/1 -> Memory1/1
  T3/1 -> Control/4(Temperature)

== system c00015M_harness/M177/Tank1 ==
  CT1 : Inport
  T1 : Inport  Port=2
  EB1 : Inport  Port=3
  LL3 : Inport  Port=4
  Control : Subsystem
  Logical Operator : Logic  AllPortsSameDT=off  OutDataTypeStr=boolean
  MasterTankControl : Subsystem
  Memory : Memory
  Memory2 : Memory
  TankModel : Subsystem
  LL1 : Outport
  wires:
  TankModel/1(LiquidLevel) -> Memory/1, LL1/1
  Control/1(LiquidIn) -> Logical Operator/1
  Control/2(LiquidOut) -> TankModel/2(LiquidOut)
  Memory/1 -> Control/5(LiquidLevel), MasterTankControl/1(LiquidTank1)
  CT1/1 -> Control/2(StartMaintenance), Control/1(ControlType)
  LL3/1 -> Memory2/1
  Memory2/1 -> MasterTankControl/2(LiquidTank3)
  EB1/1 -> Control/3(EmergencyButton)
  MasterTankControl/1(AllowTheTankFilling) -> Logical Operator/2
  Logical Operator/1 -> TankModel/1(LiquidIn)
  T1/1 -> Control/4(Temperature)

== system c00015M_harness/M177/Tank3 ==
  CT3 : Inport
  T3 : Inport  Port=2
  EB3 : Inport  Port=3
  LL1 : Inport  Port=4
  Control : Subsystem
  Logical Operator : Logic  AllPortsSameDT=off  OutDataTypeStr=boolean
  MasterTankControl : Subsystem
  Memory : Memory
  Memory1 : Memory
  TankModel : Subsystem
  LL3 : Outport
  wires:
  TankModel/1(LiquidLevel) -> Memory/1, LL3/1
  Control/1(LiquidIn) -> Logical Operator/1
  Control/2(LiquidOut) -> TankModel/2(LiquidOut)
  Memory/1 -> MasterTankControl/2(LiquidTank3), Control/5(LiquidLevel)
  CT3/1 -> Control/2(StartMaintenance), Control/1(ControlType)
  Memory1/1 -> MasterTankControl/1(LiquidTank1)
  EB3/1 -> Control/3(EmergencyButton)
  MasterTankControl/1(AllowTheTankFilling) -> Logical Operator/2
  Logical Operator/1 -> TankModel/1(LiquidIn)
  LL1/1 -> Memory1/1
  T3/1 -> Control/4(Temperature)

== system c00015M_harness/M178/Tank1 ==
  CT1 : Inport
  T1 : Inport  Port=2
  EB1 : Inport  Port=3
  LL3 : Inport  Port=4
  Control : Subsystem
  Logical Operator : Logic  AllPortsSameDT=off  OutDataTypeStr=boolean
  MasterTankControl : Subsystem
  Memory : Memory
  Memory2 : Memory
  TankModel : Subsystem
  LL1 : Outport
  wires:
  TankModel/1(LiquidLevel) -> Memory/1, LL1/1
  Control/1(LiquidIn) -> Logical Operator/1
  Control/2(LiquidOut) -> TankModel/2(LiquidOut)
  Memory/1 -> Control/5(LiquidLevel), MasterTankControl/1(LiquidTank1)
  CT1/1 -> Control/2(StartMaintenance), Control/1(ControlType)
  LL3/1 -> Memory2/1
  Memory2/1 -> MasterTankControl/2(LiquidTank3)
  EB1/1 -> Control/3(EmergencyButton)
  MasterTankControl/1(AllowTheTankFilling) -> Logical Operator/2
  Logical Operator/1 -> TankModel/1(LiquidIn)
  T1/1 -> Control/4(Temperature)

== system c00015M_harness/M178/Tank3 ==
  CT3 : Inport
  T3 : Inport  Port=2
  EB3 : Inport  Port=3
  LL1 : Inport  Port=4
  Control : Subsystem
  Logical Operator : Logic  AllPortsSameDT=off  OutDataTypeStr=boolean
  MasterTankControl : Subsystem
  Memory : Memory
  Memory1 : Memory
  TankModel : Subsystem
  LL3 : Outport
  wires:
  TankModel/1(LiquidLevel) -> Memory/1, LL3/1
  Control/1(LiquidIn) -> Logical Operator/1
  Control/2(LiquidOut) -> TankModel/2(LiquidOut)
  Memory/1 -> MasterTankControl/2(LiquidTank3), Control/5(LiquidLevel)
  CT3/1 -> Control/2(StartMaintenance), Control/1(ControlType)
  Memory1/1 -> MasterTankControl/1(LiquidTank1)
  EB3/1 -> Control/3(EmergencyButton)
  MasterTankControl/1(AllowTheTankFilling) -> Logical Operator/2
  Logical Operator/1 -> TankModel/1(LiquidIn)
  LL1/1 -> Memory1/1
  T3/1 -> Control/4(Temperature)

== system c00015M_harness/M179/Tank1 ==
  CT1 : Inport
  T1 : Inport  Port=2
  EB1 : Inport  Port=3
  LL3 : Inport  Port=4
  Control : Subsystem
  Logical Operator : Logic  AllPortsSameDT=off  OutDataTypeStr=boolean
  MasterTankControl : Subsystem
  Memory : Memory
  Memory2 : Memory
  TankModel : Subsystem
  LL1 : Outport
  wires:
  TankModel/1(LiquidLevel) -> Memory/1, LL1/1
  Control/1(LiquidIn) -> Logical Operator/1
  Control/2(LiquidOut) -> TankModel/2(LiquidOut)
  Memory/1 -> Control/5(LiquidLevel), MasterTankControl/1(LiquidTank1)
  CT1/1 -> Control/2(StartMaintenance), Control/1(ControlType)
  LL3/1 -> Memory2/1
  Memory2/1 -> MasterTankControl/2(LiquidTank3)
  EB1/1 -> Control/3(EmergencyButton)
  MasterTankControl/1(AllowTheTankFilling) -> Logical Operator/2
  Logical Operator/1 -> TankModel/1(LiquidIn)
  T1/1 -> Control/4(Temperature)

== system c00015M_harness/M179/Tank3 ==
  CT3 : Inport
  T3 : Inport  Port=2
  EB3 : Inport  Port=3
  LL1 : Inport  Port=4
  Control : Subsystem
  Logical Operator : Logic  AllPortsSameDT=off  OutDataTypeStr=boolean
  MasterTankControl : Subsystem
  Memory : Memory
  Memory1 : Memory
  TankModel : Subsystem
  LL3 : Outport
  wires:
  TankModel/1(LiquidLevel) -> Memory/1, LL3/1
  Control/1(LiquidIn) -> Logical Operator/1
  Control/2(LiquidOut) -> TankModel/2(LiquidOut)
  Memory/1 -> MasterTankControl/2(LiquidTank3), Control/5(LiquidLevel)
  CT3/1 -> Control/2(StartMaintenance), Control/1(ControlType)
  Memory1/1 -> MasterTankControl/1(LiquidTank1)
  EB3/1 -> Control/3(EmergencyButton)
  MasterTankControl/1(AllowTheTankFilling) -> Logical Operator/2
  Logical Operator/1 -> TankModel/1(LiquidIn)
  LL1/1 -> Memory1/1
  T3/1 -> Control/4(Temperature)

== system c00015M_harness/M180/Tank1 ==
  CT1 : Inport
  T1 : Inport  Port=2
  EB1 : Inport  Port=3
  LL3 : Inport  Port=4
  Control : Subsystem
  Logical Operator : Logic  AllPortsSameDT=off  OutDataTypeStr=boolean
  MasterTankControl : Subsystem
  Memory : Memory
  Memory2 : Memory
  TankModel : Subsystem
  LL1 : Outport
  wires:
  TankModel/1(LiquidLevel) -> Memory/1, LL1/1
  Control/1(LiquidIn) -> Logical Operator/1
  Control/2(LiquidOut) -> TankModel/2(LiquidOut)
  Memory/1 -> Control/5(LiquidLevel), MasterTankControl/1(LiquidTank1)
  CT1/1 -> Control/2(StartMaintenance), Control/1(ControlType)
  LL3/1 -> Memory2/1
  Memory2/1 -> MasterTankControl/2(LiquidTank3)
  EB1/1 -> Control/3(EmergencyButton)
  MasterTankControl/1(AllowTheTankFilling) -> Logical Operator/2
  Logical Operator/1 -> TankModel/1(LiquidIn)
  T1/1 -> Control/4(Temperature)

== system c00015M_harness/M180/Tank3 ==
  CT3 : Inport
  T3 : Inport  Port=2
  EB3 : Inport  Port=3
  LL1 : Inport  Port=4
  Control : Subsystem
  Logical Operator : Logic  AllPortsSameDT=off  OutDataTypeStr=boolean
  MasterTankControl : Subsystem
  Memory : Memory
  Memory1 : Memory
  TankModel : Subsystem
  LL3 : Outport
  wires:
  TankModel/1(LiquidLevel) -> Memory/1, LL3/1
  Control/1(LiquidIn) -> Logical Operator/1
  Control/2(LiquidOut) -> TankModel/2(LiquidOut)
  Memory/1 -> MasterTankControl/2(LiquidTank3), Control/5(LiquidLevel)
  CT3/1 -> Control/2(StartMaintenance), Control/1(ControlType)
  Memory1/1 -> MasterTankControl/1(LiquidTank1)
  EB3/1 -> Control/3(EmergencyButton)
  MasterTankControl/1(AllowTheTankFilling) -> Logical Operator/2
  Logical Operator/1 -> TankModel/1(LiquidIn)
  LL1/1 -> Memory1/1
  T3/1 -> Control/4(Temperature)

== system c00015M_harness/M181/Tank1 ==
  CT1 : Inport
  T1 : Inport  Port=2
  EB1 : Inport  Port=3
  LL3 : Inport  Port=4
  Control : Subsystem
  Logical Operator : Logic  AllPortsSameDT=off  OutDataTypeStr=boolean
  MasterTankControl : Subsystem
  Memory : Memory
  Memory2 : Memory
  TankModel : Subsystem
  LL1 : Outport
  wires:
  TankModel/1(LiquidLevel) -> Memory/1, LL1/1
  Control/1(LiquidIn) -> Logical Operator/1
  Control/2(LiquidOut) -> TankModel/2(LiquidOut)
  Memory/1 -> Control/5(LiquidLevel), MasterTankControl/1(LiquidTank1)
  CT1/1 -> Control/2(StartMaintenance), Control/1(ControlType)
  LL3/1 -> Memory2/1
  Memory2/1 -> MasterTankControl/2(LiquidTank3)
  EB1/1 -> Control/3(EmergencyButton)
  MasterTankControl/1(AllowTheTankFilling) -> Logical Operator/2
  Logical Operator/1 -> TankModel/1(LiquidIn)
  T1/1 -> Control/4(Temperature)

== system c00015M_harness/M181/Tank3 ==
  CT3 : Inport
  T3 : Inport  Port=2
  EB3 : Inport  Port=3
  LL1 : Inport  Port=4
  Control : Subsystem
  Logical Operator : Logic  AllPortsSameDT=off  OutDataTypeStr=boolean
  MasterTankControl : Subsystem
  Memory : Memory
  Memory1 : Memory
  TankModel : Subsystem
  LL3 : Outport
  wires:
  TankModel/1(LiquidLevel) -> Memory/1, LL3/1
  Control/1(LiquidIn) -> Logical Operator/1
  Control/2(LiquidOut) -> TankModel/2(LiquidOut)
  Memory/1 -> MasterTankControl/2(LiquidTank3), Control/5(LiquidLevel)
  CT3/1 -> Control/2(StartMaintenance), Control/1(ControlType)
  Memory1/1 -> MasterTankControl/1(LiquidTank1)
  EB3/1 -> Control/3(EmergencyButton)
  MasterTankControl/1(AllowTheTankFilling) -> Logical Operator/2
  Logical Operator/1 -> TankModel/1(LiquidIn)
  LL1/1 -> Memory1/1
  T3/1 -> Control/4(Temperature)

== system c00015M_harness/M182/Tank1 ==
  CT1 : Inport
  T1 : Inport  Port=2
  EB1 : Inport  Port=3
  LL3 : Inport  Port=4
  Control : Subsystem
  Logical Operator : Logic  AllPortsSameDT=off  OutDataTypeStr=boolean
  MasterTankControl : Subsystem
  Memory : Memory
  Memory2 : Memory
  TankModel : Subsystem
  LL1 : Outport
  wires:
  TankModel/1(LiquidLevel) -> Memory/1, LL1/1
  Control/1(LiquidIn) -> Logical Operator/1
  Control/2(LiquidOut) -> TankModel/2(LiquidOut)
  Memory/1 -> Control/5(LiquidLevel), MasterTankControl/1(LiquidTank1)
  CT1/1 -> Control/2(StartMaintenance), Control/1(ControlType)
  LL3/1 -> Memory2/1
  Memory2/1 -> MasterTankControl/2(LiquidTank3)
  EB1/1 -> Control/3(EmergencyButton)
  MasterTankControl/1(AllowTheTankFilling) -> Logical Operator/2
  Logical Operator/1 -> TankModel/1(LiquidIn)
  T1/1 -> Control/4(Temperature)

== system c00015M_harness/M182/Tank3 ==
  CT3 : Inport
  T3 : Inport  Port=2
  EB3 : Inport  Port=3
  LL1 : Inport  Port=4
  Control : Subsystem
  Logical Operator : Logic  AllPortsSameDT=off  OutDataTypeStr=boolean
  MasterTankControl : Subsystem
  Memory : Memory
  Memory1 : Memory
  TankModel : Subsystem
  LL3 : Outport
  wires:
  TankModel/1(LiquidLevel) -> Memory/1, LL3/1
  Control/1(LiquidIn) -> Logical Operator/1
  Control/2(LiquidOut) -> TankModel/2(LiquidOut)
  Memory/1 -> MasterTankControl/2(LiquidTank3), Control/5(LiquidLevel)
  CT3/1 -> Control/2(StartMaintenance), Control/1(ControlType)
  Memory1/1 -> MasterTankControl/1(LiquidTank1)
  EB3/1 -> Control/3(EmergencyButton)
  MasterTankControl/1(AllowTheTankFilling) -> Logical Operator/2
  Logical Operator/1 -> TankModel/1(LiquidIn)
  LL1/1 -> Memory1/1
  T3/1 -> Control/4(Temperature)

== system c00015M_harness/M183/Tank1 ==
  CT1 : Inport
  T1 : Inport  Port=2
  EB1 : Inport  Port=3
  LL3 : Inport  Port=4
  Control : Subsystem
  Logical Operator : Logic  AllPortsSameDT=off  OutDataTypeStr=boolean
  MasterTankControl : Subsystem
  Memory : Memory
  Memory2 : Memory
  TankModel : Subsystem
  LL1 : Outport
  wires:
  TankModel/1(LiquidLevel) -> Memory/1, LL1/1
  Control/1(LiquidIn) -> Logical Operator/1
  Control/2(LiquidOut) -> TankModel/2(LiquidOut)
  Memory/1 -> Control/5(LiquidLevel), MasterTankControl/1(LiquidTank1)
  CT1/1 -> Control/2(StartMaintenance), Control/1(ControlType)
  LL3/1 -> Memory2/1
  Memory2/1 -> MasterTankControl/2(LiquidTank3)
  EB1/1 -> Control/3(EmergencyButton)
  MasterTankControl/1(AllowTheTankFilling) -> Logical Operator/2
  Logical Operator/1 -> TankModel/1(LiquidIn)
  T1/1 -> Control/4(Temperature)

== system c00015M_harness/M183/Tank3 ==
  CT3 : Inport
  T3 : Inport  Port=2
  EB3 : Inport  Port=3
  LL1 : Inport  Port=4
  Control : Subsystem
  Logical Operator : Logic  AllPortsSameDT=off  OutDataTypeStr=boolean
  MasterTankControl : Subsystem
  Memory : Memory
  Memory1 : Memory
  TankModel : Subsystem
  LL3 : Outport
  wires:
  TankModel/1(LiquidLevel) -> Memory/1, LL3/1
  Control/1(LiquidIn) -> Logical Operator/1
  Control/2(LiquidOut) -> TankModel/2(LiquidOut)
  Memory/1 -> MasterTankControl/2(LiquidTank3), Control/5(LiquidLevel)
  CT3/1 -> Control/2(StartMaintenance), Control/1(ControlType)
  Memory1/1 -> MasterTankControl/1(LiquidTank1)
  EB3/1 -> Control/3(EmergencyButton)
  MasterTankControl/1(AllowTheTankFilling) -> Logical Operator/2
  Logical Operator/1 -> TankModel/1(LiquidIn)
  LL1/1 -> Memory1/1
  T3/1 -> Control/4(Temperature)
